simulink model "DATCOM_Forces_Moments"  (R2016b)
settings: Solver=VariableStepAuto  StartTime=0.0  StopTime=10.0  RelTol=1e-3
libraries: aerolibadyn x11, aerolibadynsys x3
settings Model: Creator=sork9  LastModifiedBy=sork9

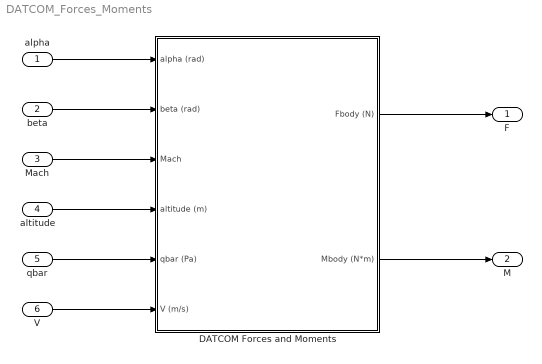
== system DATCOM_Forces_Moments ==
  alpha : Inport  Unit=rad
  beta : Inport  Port=2  Unit=rad
  Mach : Inport  Port=3  Unit=1
  altitude : Inport  Port=4  Unit=m
  qbar : Inport  Port=5  Unit=Pa
  V : Inport  Port=6  Unit=m/s
  DATCOM Forces and Moments : Subsystem
  F : Outport  Unit=N
  M : Outport  Port=2  Unit=N*m
  wires:
  alpha/1 -> DATCOM Forces and Moments/1(alpha (rad))
  beta/1 -> DATCOM Forces and Moments/2(beta (rad))
  Mach/1 -> DATCOM Forces and Moments/3(Mach)
  altitude/1 -> DATCOM Forces and Moments/4(altitude (m))
  qbar/1 -> DATCOM Forces and Moments/5(qbar (Pa))
  V/1 -> DATCOM Forces and Moments/6(V (m/s))
  DATCOM Forces and Moments/1(Fbody (N)) -> F/1
  DATCOM Forces and Moments/2(Mbody (N*m)) -> M/1

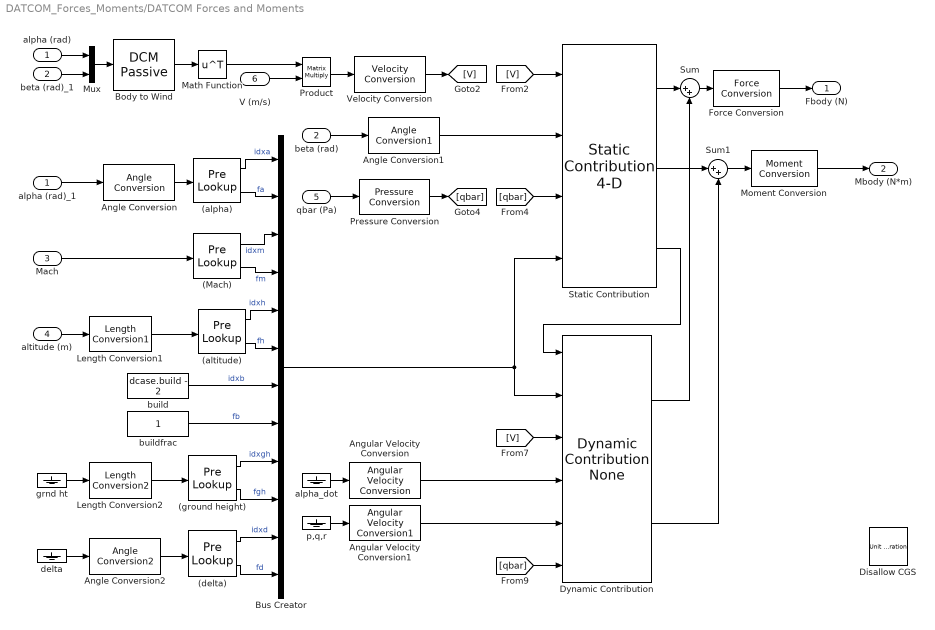
== system DATCOM_Forces_Moments/DATCOM Forces and Moments ==
  alpha (rad) : Inport  Unit=rad
  beta (rad) : Inport  Port=2  Unit=rad
  Mach : Inport  Port=3  Unit=1
  altitude (m) : Inport  Port=4  Unit=m
  qbar (Pa) : Inport  Port=5  Unit=Pa
  V (m/s) : Inport  Port=6  Unit=m/s
  (Mach) : PreLookup  BreakpointsData=0:2  BeginIndexSearchUsingPreviousIndexResult=on  IndexDataTypeStr=int32  FractionDataTypeStr=double
  (alpha) : PreLookup  BreakpointsData=dcase.alpha  BeginIndexSearchUsingPreviousIndexResult=on  IndexDataTypeStr=int32  FractionDataTypeStr=double
  (altitude) : PreLookup  BreakpointsData=0:2  BeginIndexSearchUsingPreviousIndexResult=on  IndexDataTypeStr=int32  FractionDataTypeStr=double
  (delta) : PreLookup  BreakpointsData=[0:2]  BeginIndexSearchUsingPreviousIndexResult=on  IndexDataTypeStr=int32  FractionDataTypeStr=double
  (ground height) : PreLookup  BreakpointsData=[0:2]  BeginIndexSearchUsingPreviousIndexResult=on  IndexDataTypeStr=int32  FractionDataTypeStr=double
  Angle Conversion : aerolibadyn/Digital DATCOM Forces and Moments/Angle Conversion
  Angle Conversion1 : aerolibadyn/Digital DATCOM Forces and Moments/Angle Conversion1
  Angle Conversion2 : aerolibadyn/Digital DATCOM Forces and Moments/Angle Conversion2
  Angular Velocity Conversion : aerolibadyn/Digital DATCOM Forces and Moments/Angular Velocity Conversion
  Angular Velocity Conversion1 : aerolibadyn/Digital DATCOM Forces and Moments/Angular Velocity Conversion1
  Body to Wind : aerolibadynsys/DCM Passive  SystemSampleTime=-1
  Bus Creator : BusCreator  Inputs=12
  Disallow CGS : UnitConfiguration  UnitSystemsStr=English,SI,SI (extended)  AllowAllUnitSystems=off
  Dynamic Contribution : aerolibadynsys/Dynamic Contribution None  Unit=deg/s
  Force Conversion : aerolibadyn/Digital DATCOM Forces and Moments/Force Conversion
  Length Conversion1 : aerolibadyn/Digital DATCOM Forces and Moments/Length Conversion1
  Length Conversion2 : aerolibadyn/Digital DATCOM Forces and Moments/Length Conversion2
  Math Function : Math  Operator=transpose  SaturateOnIntegerOverflow=on
  Moment Conversion : aerolibadyn/Digital DATCOM Forces and Moments/Moment Conversion
  Mux : Mux  Inputs=2
  Pressure Conversion : aerolibadyn/Digital DATCOM Forces and Moments/Pressure Conversion
  Product : Product  Multiplication=Matrix(*)  RndMeth=Zero
  Static Contribution : aerolibadynsys/Static Contribution 4-D  SystemSampleTime=-1
  Sum : Sum  Inputs=|++
  Sum1 : Sum  Inputs=|++
  Velocity Conversion : aerolibadyn/Digital DATCOM Forces and Moments/Velocity Conversion
  alpha (rad)_1 : InportShadow  Unit=rad
  alpha_dot : Ground
  beta (rad)_1 : InportShadow  Port=2  Unit=rad
  build : Constant  Value=dcase.build - 2  OutDataTypeStr=int32
  buildfrac : Constant  OutDataTypeStr=double
  delta : Ground
  grnd ht : Ground
  p,q,r : Ground
  Fbody (N) : Outport  Unit=N
  Mbody (N*m) : Outport  Port=2  Unit=N*m
  wires:
  Math Function/1 -> Product/1
  V (m/s)/1 -> Product/2
  (ground height)/1 -> Bus Creator/9  "idxgh"
  Length Conversion2/1 -> (ground height)/1
  (delta)/2 -> Bus Creator/12  "fd"
  (delta)/1 -> Bus Creator/11  "idxd"
  Velocity Conversion/1 -> [V]
  Angular Velocity Conversion1/1 -> Dynamic Contribution/5
  Angular Velocity Conversion/1 -> Dynamic Contribution/4
  Pressure Conversion/1 -> [qbar]
  Moment Conversion/1 -> Mbody (N*m)/1
  Length Conversion1/1 -> (altitude)/1
  [qbar] -> Dynamic Contribution/6
  [V] -> Dynamic Contribution/3
  Dynamic Contribution/1 -> Sum/2
  qbar (Pa)/1 -> Pressure Conversion/1
  grnd ht/1 -> Length Conversion2/1
  Product/1 -> Velocity Conversion/1
  beta (rad)/1 -> Angle Conversion1/1
  alpha_dot/1 -> Angular Velocity Conversion/1
  Dynamic Contribution/2 -> Sum1/2
  Static Contribution/1 -> Sum/1
  Static Contribution/3 -> Dynamic Contribution/1
  Force Conversion/1 -> Fbody (N)/1
  Static Contribution/2 -> Sum1/1
  delta/1 -> Angle Conversion2/1
  Sum/1 -> Force Conversion/1
  altitude (m)/1 -> Length Conversion1/1
  alpha (rad)_1/1 -> Angle Conversion/1
  p,q,r/1 -> Angular Velocity Conversion1/1
  (Mach)/1 -> Bus Creator/3  "idxm"
  Angle Conversion2/1 -> (delta)/1
  Mux/1 -> Body to Wind/1
  Bus Creator/1 -> Static Contribution/4, Dynamic Contribution/2
  alpha (rad)/1 -> Mux/1
  beta (rad)_1/1 -> Mux/2
  Body to Wind/1 -> Math Function/1
  Mach/1 -> (Mach)/1
  (alpha)/1 -> Bus Creator/1  "idxa"
  (alpha)/2 -> Bus Creator/2  "fa"
  [V] -> Static Contribution/1
  Angle Conversion/1 -> (alpha)/1
  (Mach)/2 -> Bus Creator/4  "fm"
  (altitude)/2 -> Bus Creator/6  "fh"
  (altitude)/1 -> Bus Creator/5  "idxh"
  buildfrac/1 -> Bus Creator/8  "fb"
  build/1 -> Bus Creator/7  "idxb"
  Angle Conversion1/1 -> Static Contribution/2
  (ground height)/2 -> Bus Creator/10  "fgh"
  [qbar] -> Static Contribution/3
  Sum1/1 -> Moment Conversion/1
